simulink library "INT_AccPed_DrvDemLead"  (R2016b)
settings: Solver=VariableStepAuto  StartTime=0.0  StopTime=10.0  RelTol=1e-3
settings Model: Creator=bianxuyin  LastModifiedBy=bianxuyin

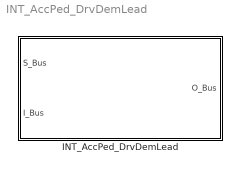
== system INT_AccPed_DrvDemLead ==
  INT_AccPed_DrvDemLead : Subsystem

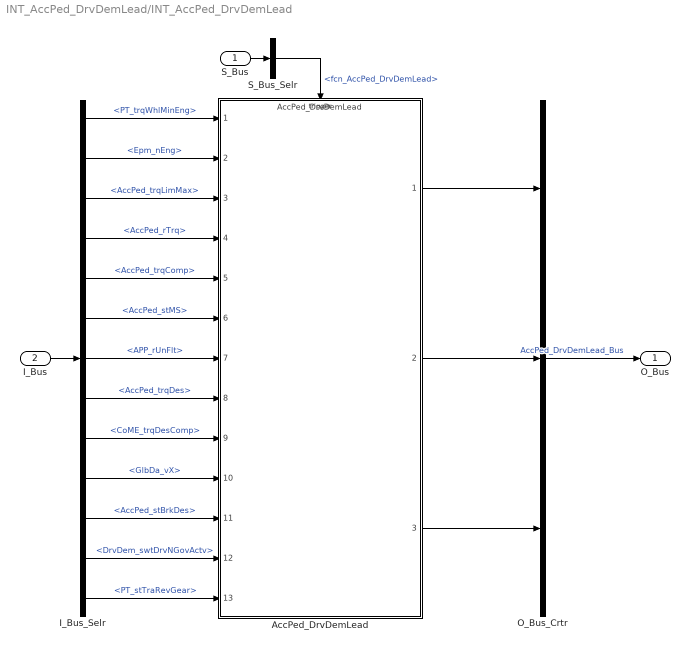
== system INT_AccPed_DrvDemLead/INT_AccPed_DrvDemLead ==
  S_Bus : Inport
  I_Bus : Inport  Port=2
  AccPed_DrvDemLead : ModelReference  ModelNameDialog=AccPed_DrvDemLead  SimulationMode=Normal  ModelReferenceVersion=1.29  TriggerPortName=function  TriggerPortTriggerType=function-call  TriggerPortStatesWhenEnabling=held
  I_Bus_Selr : BusSelector  OutputSignals=PT_trqWhlMinEng,Epm_nEng,AccPed_trqLimMax,AccPed_rTrq,AccPed_trqComp,AccPed_stMS,APP_rUnFlt,AccPed_trqDes,CoME_trqDesComp,GlbDa_vX,AccPed_stBrkDes,DrvDem_swtDrvNGovActv,PT_stTraRevGear
  O_Bus_Crtr : BusCreator  Inputs=3
  S_Bus_Selr : BusSelector  OutputSignals=fcn_AccPed_DrvDemLead
  O_Bus : Outport
  wires:
  S_Bus_Selr/1 -> AccPed_DrvDemLead/Trigger  "<fcn_AccPed_DrvDemLead>"
  S_Bus/1 -> S_Bus_Selr/1
  I_Bus/1 -> I_Bus_Selr/1
  I_Bus_Selr/1 -> AccPed_DrvDemLead/1  "<PT_trqWhlMinEng>"
  I_Bus_Selr/2 -> AccPed_DrvDemLead/2  "<Epm_nEng>"
  I_Bus_Selr/3 -> AccPed_DrvDemLead/3  "<AccPed_trqLimMax>"
  I_Bus_Selr/4 -> AccPed_DrvDemLead/4  "<AccPed_rTrq>"
  I_Bus_Selr/5 -> AccPed_DrvDemLead/5  "<AccPed_trqComp>"
  I_Bus_Selr/6 -> AccPed_DrvDemLead/6  "<AccPed_stMS>"
  I_Bus_Selr/7 -> AccPed_DrvDemLead/7  "<APP_rUnFlt>"
  I_Bus_Selr/8 -> AccPed_DrvDemLead/8  "<AccPed_trqDes>"
  I_Bus_Selr/9 -> AccPed_DrvDemLead/9  "<CoME_trqDesComp>"
  I_Bus_Selr/10 -> AccPed_DrvDemLead/10  "<GlbDa_vX>"
  I_Bus_Selr/11 -> AccPed_DrvDemLead/11  "<AccPed_stBrkDes>"
  I_Bus_Selr/12 -> AccPed_DrvDemLead/12  "<DrvDem_swtDrvNGovActv>"
  I_Bus_Selr/13 -> AccPed_DrvDemLead/13  "<PT_stTraRevGear>"
  O_Bus_Crtr/1 -> O_Bus/1  "AccPed_DrvDemLead_Bus"
  AccPed_DrvDemLead/1 -> O_Bus_Crtr/1
  AccPed_DrvDemLead/2 -> O_Bus_Crtr/2
  AccPed_DrvDemLead/3 -> O_Bus_Crtr/3
